simulink model "q4_3_impulse"  (R2023a)
settings: Solver=VariableStepAuto  StartTime=0.0  StopTime=20.0  RelTol=1e-3
libraries: dspsrcs4 x2, simulink x1
settings Model: Creator=user  LastModifiedBy=user

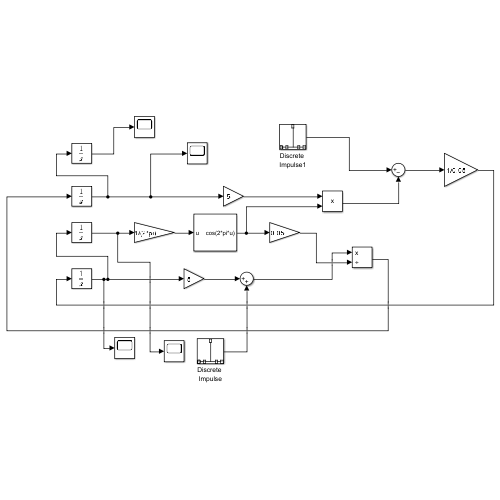
[thumbnail: Simulink's stored preview of the top-level diagram]
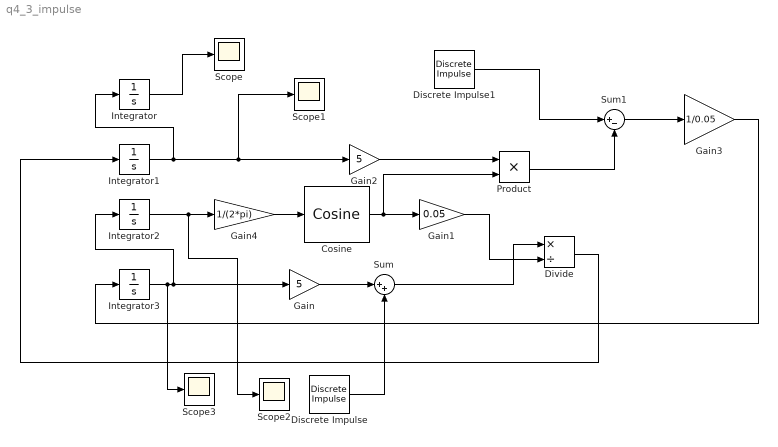
== system q4_3_impulse ==
  Cosine : simulink/Lookup Tables/Cosine  Formula=cos(2*pi*u)  NumDataPoints=(2^5)+1  OutputWordLength=16  InternalRulePriority=Speed
  Discrete Impulse : dspsrcs4/Discrete  Impulse  Delay=0  SampleTime=1  FrameSample=1  OutputFrames=off  dataType=double  isSigned=on  wordLen=16  udDataType=sfix(16)  fracBitsMode=Best precision  numFracBits=15  OutDataTypeStr=double  LastOutDataTypeStr=double
  Discrete Impulse1 : dspsrcs4/Discrete  Impulse  Delay=0  SampleTime=1  FrameSample=1  OutputFrames=off  dataType=double  isSigned=on  wordLen=16  udDataType=sfix(16)  fracBitsMode=Best precision  numFracBits=15  OutDataTypeStr=double  LastOutDataTypeStr=double
  Divide : Product  Inputs=*/  OutMin=[0.001]
  Gain : Gain  Gain=5
  Gain1 : Gain  Gain=0.05
  Gain2 : Gain  Gain=5
  Gain3 : Gain  Gain=1/0.05
  Gain4 : Gain  Gain=1/(2*pi)
  Integrator{,1..3} (4 alike) : Integrator
  Product : Product
  Scope{,1..3} (4 alike) : Scope
  Sum : Sum  Inputs=|++
  Sum1 : Sum  Inputs=|+-
  wires:
  Integrator1/1 -> Scope1/1, Gain2/1, Integrator/1
  Integrator3/1 -> Gain/1, Integrator2/1, Scope3/1
  Gain/1 -> Sum/1
  Cosine/1 -> Product/2, Gain1/1
  Gain1/1 -> Divide/2
  Sum/1 -> Divide/1
  Divide/1 -> Integrator1/1
  Gain2/1 -> Product/1
  Product/1 -> Sum1/2
  Sum1/1 -> Gain3/1
  Gain3/1 -> Integrator3/1
  Gain4/1 -> Cosine/1
  Integrator2/1 -> Scope2/1, Gain4/1
  Integrator/1 -> Scope/1
  Discrete Impulse/1 -> Sum/2
  Discrete Impulse1/1 -> Sum1/1
